simulink model "int_dezim1"  (Simulink 7.8)
settings: Solver=FixedStepDiscrete  SolverMode=SingleTasking  StartTime=0.0  StopTime=1  RelTol=1e-3
libraries: dspmlti4 x2, simulink x1, dspsigops x1
settings Model: Creator=svenhoffmann  LastModifiedBy=josef  ExtModeAutoUpdateStatusClock=off
settings DataIOCC: SignalLoggingName=sigsOut
settings OptimizationCC: InitFltsAndDblsToZero=on
settings DebuggingCC: SaveWithParameterizedLinksMsg=none  SignalResolutionControl=TryResolveAllWithWarning  SolverPrmCheckMsg=none  MultiTaskDSMMsg=warning  MultiTaskCondExecSysMsg=none  FcnCallInpInsideContextMsg=Use local settings  StrictBusMsg=None
settings HardwareCC: TargetUnknown=on
settings RTWCC: IncludeERTFirstTime=on
settings GRTTargetCC: TargetFcnLib=ansi_tfl_tmw.mat

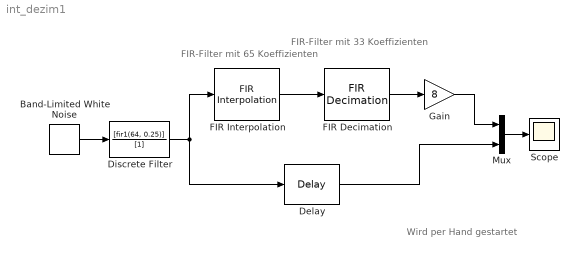
== system int_dezim1 ==
  note: FIR-Filter
      | mit 65 Koeffizienten
  note: FIR-Filter
      | mit 33 Koeffizienten
  note: Wird per Hand gestartet
  Band-Limited White Noise : simulink/Sources/Band-Limited White Noise  Cov=[1/1000]  Ts=1/1000  seed=[23341]
  Delay : dspsigops/Delay  InputProcessing=Inherited (this choice will be removed - see release notes)  dly_unit=Samples  delay=6  ic_detail=off  dif_ic_for_ch=off  dif_ic_for_dly=off  ic=0  reset_popup=None
  Discrete Filter : DiscreteFilter  Numerator=[fir1(64, 0.25)]  Denominator=[1]  SampleTime=1/1000
  FIR Decimation : dspmlti4/FIR Decimation  h=fir1(32,1/3)  D=3  filtStruct=Direct form  framing=Maintain input frame size  inputOffset=0  outputBufInitCond=0  InputProcessing=Inherited (this choice will be removed - see release notes)  firstCoeffDataTypeStr=Inherit: Same word length as input  firstCoeffLastDataTypeStr=Inherit: Same word length as input  firstCoeffMin=[]  firstCoeffMax=[]  outputMin=[]  outputMax=[]  roundingMode=Floor  overflowMode=off  FilterSource=Specify via dialog  FilterObject=Hm_firdecim
  FIR Interpolation : dspmlti4/FIR Interpolation  h=fir1(64,1/8)  L=8  framing=Maintain input frame size  outputBufInitCond=0  InputProcessing=Inherited (this choice will be removed - see release notes)  firstCoeffDataTypeStr=Inherit: Same word length as input  firstCoeffLastDataTypeStr=Inherit: Same word length as input  firstCoeffMin=[]  firstCoeffMax=[]  outputMin=[]  outputMax=[]  roundingMode=Floor  overflowMode=off  FilterSource=Specify via dialog  FilterObject=Hm_firinterp
  Gain : Gain  Gain=8  SaturateOnIntegerOverflow=on  OutDataTypeStr=Inherit: Same as input  ParamDataTypeStr=Inherit: Same as input
  Mux : Mux  Inputs=2
  Scope : Scope
  wires:
  FIR Interpolation/1 -> FIR Decimation/1
  Band-Limited White Noise/1 -> Discrete Filter/1
  Discrete Filter/1 -> FIR Interpolation/1, Delay/1
  FIR Decimation/1 -> Gain/1
  Delay/1 -> Mux/2
  Mux/1 -> Scope/1
  Gain/1 -> Mux/1
